simulink model "on_grid_new"  (R2015b)
settings: Solver=VariableStepAuto  StartTime=0.0  StopTime=5  RelTol=1e-3
undefined symbols (not defined in the file): Ts_Control, Ts_Power
libraries: powerlib x41, powerlib_meascontrol x16, simulink x3, powerlib_extras x1
settings Model: Creator=fujitsu  LastModifiedBy=fujitsu

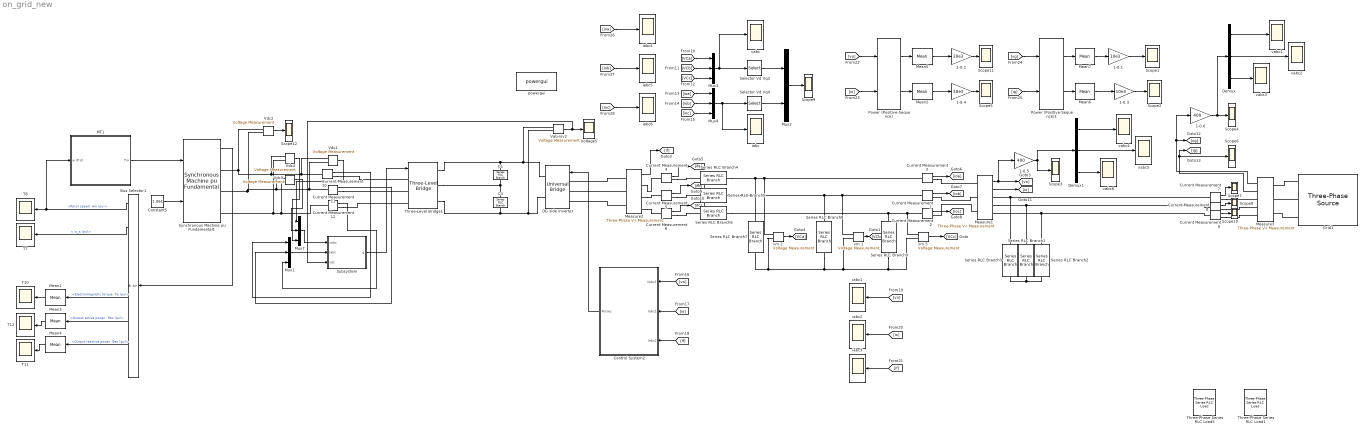
== system on_grid_new ==
  1-0.1 : Gain  Gain=10e3
  1-0.2 : Gain  Gain=30e3
  1-0.3 : Gain  Gain=10e3
  1-0.4 : Gain  Gain=30e3
  1-0.5 : Gain  Gain=400
  1-0.6 : Gain  Gain=400
  Bus Selector1 : BusSelector  OutputSignals="Mechanical.Rotor speed  wm (pu),Stator current. is_a (pu),Stator current. is_b (pu),Stator current. is_c (pu),Mechanical.Electromagnetic torque  Te (pu),Output active power   Peo (pu),Output reactive power  Qeo (pu),Mechanical.Rotor mechanical angle  theta (deg)"
  C1 : powerlib/Elements/Series RLC Branch  LConnTagsString=__new0  RConnTagsString=__new0  BranchType=C  Resistance=1.0  Inductance=1.0  SetiL0=off  InitialCurrent=0  Capacitance=5000e-06  Setx0=off  InitialVoltage=0  Measurements=None
  C3 : powerlib/Elements/Series RLC Branch  LConnTagsString=__new0  RConnTagsString=__new0  BranchType=C  Resistance=1.0  Inductance=1.0  SetiL0=off  InitialCurrent=0  Capacitance=5000e-06  Setx0=off  InitialVoltage=0  Measurements=None
  Constant5 : Constant  Value=1.061
  Control System2 : Subsystem
  Current Measurement{1..12} (12 alike) : powerlib/Measurements/Current Measurement  PhasorSimulation=off  OutputType=Complex  PSBequivalent=0
  DG side Inverter : powerlib/Power Electronics/Universal Bridge  Arms=3  SnubberResistance=10000  SnubberCapacitance=inf  Device=IGBT / Diodes  Ron=1e-4  Lon=0  ForwardVoltages="[  1  1  ]"  ForwardVoltage=.8  GTOparameters=[ 10e-6 , 20e-6 ]  IGBTparameters=[ 1e-6 , 2e-6 ]  Measurements=None  Measurements_2=None  converterType=Rectifier
  Demux : Demux  Outputs=3
  Demux1 : Demux  Outputs=3
  Grid1 : powerlib/Electrical Sources/Three-Phase Source  InternalConnection=Yg  VoltagePhases=off  Voltage=400  PhaseAngle=0  Voltage_phases=[25e3 25e3 25e3]/sqrt(3)  PhaseAngles_phases=[0 -120 +120]  Frequency=50  NonIdealSource=on  SpecifyImpedance=off  Resistance=0.02  Inductance=0.3e-3  ShortCircuitLevel=100e6  BaseVoltage=60e3  XRratio=1  BusType=swing  Pref=0  Qref=0  Prefabc=[10e3, 10e3, 10e3]  Qrefabc=[0, 0, 0]  Qmin=-inf  Qmax=inf
  MT1 : Subsystem
  Mean{1..7} (7 alike) : powerlib_meascontrol/Measurements/Mean  Freq=50  Vinit=0  Ts=5e-6
  Measure1 : powerlib/Measurements/Three-Phase V-I Measurement  VoltageMeasurement=phase-to-ground  SetLabelV=off  LabelV=V1  Vpu=on  VpuLL=off  CurrentMeasurement=yes  SetLabelI=off  LabelI=I1  Ipu=on  Pbase=30e3  Vbase=400  OutputType=Magnitude  PhasorSimulation=off  PSBequivalent=0
  Measure2 : powerlib/Measurements/Three-Phase V-I Measurement  VoltageMeasurement=no  SetLabelV=off  LabelV=V1  Vpu=off  VpuLL=off  CurrentMeasurement=yes  SetLabelI=off  LabelI=I1  Ipu=on  Pbase=30e3  Vbase=400  OutputType=Magnitude  PhasorSimulation=off  PSBequivalent=0
  Measure3 : powerlib/Measurements/Three-Phase V-I Measurement  VoltageMeasurement=phase-to-ground  SetLabelV=off  LabelV=V1  Vpu=on  VpuLL=off  CurrentMeasurement=yes  SetLabelI=off  LabelI=I1  Ipu=on  Pbase=10e3  Vbase=400  OutputType=Magnitude  PhasorSimulation=off  PSBequivalent=0
  Mux{1,3..4,7} (4 alike) : Mux  Inputs=3
  Mux2 : Mux  Inputs=2
  Power (Positive-Sequence) : powerlib_meascontrol/Measurements/Power (Positive-Sequence)  Freq=50  Vinit=[0, 0]  Iinit=[0, 0]  Ts=5e-6
  Power (Positive-Sequence)1 : powerlib_meascontrol/Measurements/Power (Positive-Sequence)  Freq=50  Vinit=[0, 0]  Iinit=[0, 0]  Ts=5e-6
  Scope{1..12} (12 alike) : Scope
  Selector Vd Vq3 : Selector  InputPortWidth=3  IndexOptions=Index vector (dialog)  Indices=[1]  OutputSizes=1
  Selector Vd Vq4 : Selector  InputPortWidth=3  IndexOptions=Index vector (dialog)  Indices=[1]  OutputSizes=1
  Series RLC Branch1 : powerlib/Elements/Series RLC Branch  LConnTagsString=__new0  RConnTagsString=__new0  BranchType=RL  Resistance=50*0.5  Inductance=100e-3*0.5  SetiL0=off  InitialCurrent=0  Capacitance=1e-6  Setx0=off  InitialVoltage=0  Measurements=None
  Series RLC Branch2 : powerlib/Elements/Series RLC Branch  LConnTagsString=__new0  RConnTagsString=__new0  BranchType=RL  Resistance=50*0.5  Inductance=100e-3*0.5  SetiL0=off  InitialCurrent=0  Capacitance=1e-6  Setx0=off  InitialVoltage=0  Measurements=None
  Series RLC Branch3 : powerlib/Elements/Series RLC Branch  LConnTagsString=__new0  RConnTagsString=__new0  BranchType=RL  Resistance=50*0.5  Inductance=100e-3*0.5  SetiL0=off  InitialCurrent=0  Capacitance=1e-6  Setx0=off  InitialVoltage=0  Measurements=None
  Series RLC Branch4 : powerlib/Elements/Series RLC Branch  LConnTagsString=__new0  RConnTagsString=__new0  BranchType=L  Resistance=5  Inductance=3e-3  SetiL0=off  InitialCurrent=0  Capacitance=1e-6  Setx0=off  InitialVoltage=0  Measurements=None
  Series RLC Branch5 : powerlib/Elements/Series RLC Branch  LConnTagsString=__new0  RConnTagsString=__new0  BranchType=L  Resistance=5  Inductance=3e-3  SetiL0=off  InitialCurrent=0  Capacitance=1e-6  Setx0=off  InitialVoltage=0  Measurements=None
  Series RLC Branch6 : powerlib/Elements/Series RLC Branch  LConnTagsString=__new0  RConnTagsString=__new0  BranchType=L  Resistance=5  Inductance=3e-3  SetiL0=off  InitialCurrent=0  Capacitance=1e-6  Setx0=off  InitialVoltage=0  Measurements=None
  Series RLC Branch7 : powerlib/Elements/Series RLC Branch  LConnTagsString=__new0  RConnTagsString=__new0  BranchType=C  Resistance=5  Inductance=10e-3  SetiL0=off  InitialCurrent=0  Capacitance=300e-6  Setx0=off  InitialVoltage=0  Measurements=None
  Series RLC Branch8 : powerlib/Elements/Series RLC Branch  LConnTagsString=__new0  RConnTagsString=__new0  BranchType=C  Resistance=5  Inductance=10e-3  SetiL0=off  InitialCurrent=0  Capacitance=300e-6  Setx0=off  InitialVoltage=0  Measurements=None
  Series RLC Branch9 : powerlib/Elements/Series RLC Branch  LConnTagsString=__new0  RConnTagsString=__new0  BranchType=C  Resistance=5  Inductance=10e-3  SetiL0=off  InitialCurrent=0  Capacitance=300e-6  Setx0=off  InitialVoltage=0  Measurements=None
  Subsystem : Subsystem  mask{kp=0.0001, ki=5, dcref=750}
      mask prompts: dcref "Vdc_ref"
  Synchronous Machine pu Fundamental1 : powerlib/Machines/Synchronous Machine pu Fundamental  PresetModel=No  MechanicalLoad=Mechanical power Pm  ShowDetailedParameters=on  RotorType=Salient-pole  Units=per unit fundamental parameters  MeasurementBus=off  NominalParameters="[ 30e3  550 1600]"  Stator="[ 0.2503  0.114  0.6875  0.6875 ]"  Field="[ 1  10e15/(100*pi)]"  Dampers2=[0.0652, 0.5134, 0.0287, 0.2553, 7.765e-3, 0.9167 ]  Dampers1="[ 1.17E-02  0.182  1.97E-02  0.384 ]"  Mechanical=[ 6 0 2]  PolePairs=20  InitialConditions="[ 0  0  0  0  0  0  0  0  1 ]"  SetSaturation=off  Saturation=[0.6404,0.7127,0.8441,0.9214,0.9956,1.082,1.19,1.316,1.457;0.7,0.7698,0.8872,0.9466,0.9969,1.046,1.1,1.151,1.201]  LoadFlowParameters=[1,0,0,0,0]  TsPowergui=0  TsBlock=-1  IterativeModel=Trapezoidal non iterative  BusType=swing  Pref=0  Qref=0  Qmin=-inf  Qmax=inf  PLF=0  QLF=0
  T{7..8,10..12} (5 alike) : Scope
  Three-Level Bridge1 : powerlib/Power Electronics/Three-Level Bridge  Arms=3  SnubberResistance=100  SbubberCapacitance=1e-6  Device=IGBT / Diodes  Ron=1e-3  ForwardVoltages=[350 1]  Measurements=All voltages and currents
  Three-Phase Series RLC Load1 : powerlib/Elements/Three-Phase Series RLC Load  LConnTagsString=A|B|C  Configuration=Y (grounded)  NominalVoltage=400  Vabc=[1e3 1e3 1e3]  Vabcp=[1e3 1e3 1e3]  NominalFrequency=50  UnbalancedPower=off  ActivePower=50e3  InductivePower=0  CapacitivePower=0  Pabc=[10e3 9e3 11e3]  QLabc=[100 90 110]  QCabc=[100 90 110]  Pabcp=[10e3 9e3 11e3]  QLabcp=[100 90 110]  QCabcp=[100 90 110]  Measurements=None  LoadType=constant Z
  Three-Phase Series RLC Load5 : powerlib/Elements/Three-Phase Series RLC Load  LConnTagsString=A|B|C  Configuration=Y (grounded)  NominalVoltage=400  Vabc=[1e3 1e3 1e3]  Vabcp=[1e3 1e3 1e3]  NominalFrequency=50  UnbalancedPower=off  ActivePower=50e3  InductivePower=0  CapacitivePower=0  Pabc=[10e3 9e3 11e3]  QLabc=[100 90 110]  QCabc=[100 90 110]  Pabcp=[10e3 9e3 11e3]  QLabcp=[100 90 110]  QCabcp=[100 90 110]  Measurements=None  LoadType=constant Z
  Vab-inv2 : powerlib/Measurements/Voltage Measurement  Tag=PoWeRsYsTeMmEaSuReMeNt  PhasorSimulation=off  OutputType=Magnitude  PSBequivalent=0
  Vdc{1..4} (4 alike) : powerlib/Measurements/Voltage Measurement  Tag=PoWeRsYsTeMmEaSuReMeNt  PhasorSimulation=off  OutputType=Magnitude  PSBequivalent=0
  Voltage5 : Scope
  iabc{,1..6} (7 alike) : Scope
  powergui : powerlib/powergui  SimulationMode=Discrete  SolverType=Tustin  SampleTime=5e-6  frequency=60  SPID=off  DisableSnubberDevices=off  DisableRonSwitches=off  DisableVfSwitches=off  SwTol=0  DisplayEquations=off  Interpol=off  ExternalGateDelay=off  methode=off  Ts=0  FunctionMessages=off  echomessages=off  HookPort=off  EnableUseOfTLC=off  x0status=blocks  frequencyindice=0  Pbase=100e6  ErrMax=0.0001  Iterations=50  UnitsV=kV  UnitsW=MW  buscounter=0  RestoreLinks=warning  ResistiveCurrentMeasurement=off  Frange=[0:2:500]  Ylog=off  Xlog=on  ShowGrid=off  save=off  variable=ZData  structure=Vs  ZoomFFT=on  StartTime=1/60  cycles=1  DisplayStyle=1  fundamental=60  FreqAxis=on  MaxFrequency=10000  frequencyindicesteady=1  RmsSteady=1  display=off
  vabc{,1..6} (7 alike) : Scope
  vm 1 : powerlib/Measurements/Voltage Measurement  PhasorSimulation=off  OutputType=Complex  PSBequivalent=0
  vm 2 : powerlib/Measurements/Voltage Measurement  PhasorSimulation=off  OutputType=Complex  PSBequivalent=0
  vm 5 : powerlib/Measurements/Voltage Measurement  PhasorSimulation=off  OutputType=Complex  PSBequivalent=0
  wires:
  Control System2/1(Pulses) -> DG side Inverter/1
  vm 5/1 -> [VCc]
  vm 1/1 -> [VCb]
  vm 2/1 -> [VCa]
  Current Measurement2/1 -> [ioc]
  Current Measurement1/1 -> [iob]
  Current Measurement3/1 -> [ioa]
  Current Measurement4/1 -> [ifa]
  Current Measurement5/1 -> [ifb]
  Current Measurement6/1 -> [ifc]
  Power (Positive-Sequence)/1 -> Mean5/1
  Mux2/1 -> Scope9/1
  Selector Vd Vq3/1 -> Mux2/1
  Selector Vd Vq4/1 -> Mux2/2
  Power (Positive-Sequence)/2 -> Mean2/1
  [VCc] -> Mux3/3
  [VCa] -> Mux3/1
  [VCb] -> Mux3/2
  Mux3/1 -> Selector Vd Vq3/1, vabc/1
  [ioa] -> Mux4/1
  [iob] -> Mux4/2
  [ioc] -> Mux4/3
  Mux4/1 -> Selector Vd Vq4/1, iabc/1
  Measure2/1 -> [if]
  Measure1/1 -> 1-0.5/1, [vo]
  Measure1/2 -> [io]
  [vo] -> Control System2/1(Vabc1)
  [vo] -> iabc1/1
  [io] -> iabc2/1
  [if] -> iabc3/1
  Measure3/1 -> 1-0.6/1, [vg]
  Measure3/2 -> [ig], Scope6/1
  Power (Positive-Sequence)1/1 -> Mean7/1
  Power (Positive-Sequence)1/2 -> Mean6/1
  [vg] -> Power (Positive-Sequence)1/1
  [ig] -> Power (Positive-Sequence)1/2
  Mean7/1 -> 1-0.1/1
  Mean6/1 -> 1-0.3/1
  1-0.3/1 -> Scope2/1
  1-0.1/1 -> Scope1/1
  1-0.2/1 -> Scope11/1
  Mean5/1 -> 1-0.2/1
  1-0.4/1 -> Scope5/1
  Mean2/1 -> 1-0.4/1
  [io] -> Control System2/2(Iabc1)
  [if] -> Control System2/3(Iabc2)
  1-0.5/1 -> Demux1/1, Scope3/1
  1-0.6/1 -> Demux/1, Scope4/1
  [ioa] -> iabc4/1
  [iob] -> iabc5/1
  [ioc] -> iabc6/1
  Demux/3 -> vabc3/1
  Demux/2 -> vabc2/1
  Demux/1 -> vabc1/1
  [vo] -> Power (Positive-Sequence)/1
  [io] -> Power (Positive-Sequence)/2
  Demux1/3 -> vabc6/1
  Demux1/2 -> vabc5/1
  Demux1/1 -> vabc4/1
  Current Measurement7/1 -> Scope7/1
  Current Measurement8/1 -> Scope8/1
  Current Measurement9/1 -> Scope10/1
  MT1/1(Tm) -> Synchronous Machine pu Fundamental1/1
  Synchronous Machine pu Fundamental1/1 -> Bus Selector1/1
  Constant5/1 -> Synchronous Machine pu Fundamental1/2
  Vdc2/1 -> Scope12/1
  Vab-inv2/1 -> Subsystem/3(vdc), Voltage5/1
  Mean4/1 -> T11/1
  Bus Selector1/1 -> MT1/1(w (P.U)), T8/1  "<Rotor speed  wm (pu)>"
  Bus Selector1/5 -> Mean1/1  "<Electromagnetic torque  Te (pu)>"
  Mean1/1 -> T10/1
  Bus Selector1/7 -> Mean4/1  "<Output reactive power  Qeo (pu)>"
  Bus Selector1/6 -> Mean3/1  "<Output active power   Peo (pu)>"
  Mean3/1 -> T12/1
  Bus Selector1/2 -> T7/1  "< is_a (pu)>"
  Subsystem/1(g) -> Three-Level Bridge1/1
  Current Measurement10/1 -> Mux1/1
  Current Measurement11/1 -> Mux1/2
  Current Measurement12/1 -> Mux1/3
  Mux1/1 -> Subsystem/2(Iabc)
  Vdc1/1 -> Mux7/1
  Vdc3/1 -> Mux7/2
  Vdc4/1 -> Mux7/3
  Mux7/1 -> Subsystem/1(vabc)
  connections:
  C3/RConn1 -- Three-Level Bridge1/RConn3 -- DG side Inverter/RConn2 -- Vab-inv2/LConn2
  Three-Level Bridge1/RConn1 -- C1/LConn1 -- DG side Inverter/RConn1 -- Vab-inv2/LConn1
  Series RLC Branch7/LConn1 -- Series RLC Branch4/RConn1 -- Current Measurement3/LConn1 -- vm 2/LConn1
  Current Measurement1/LConn1 -- vm 1/LConn1 -- Series RLC Branch5/RConn1 -- Series RLC Branch8/LConn1
  Series RLC Branch9/LConn1 -- Series RLC Branch6/RConn1 -- Current Measurement2/LConn1 -- vm 5/LConn1
  vm 2/LConn2 -- Series RLC Branch7/RConn1 -- Series RLC Branch8/RConn1 -- vm 1/LConn2 -- Series RLC Branch9/RConn1 -- vm 5/LConn2
  Measure1/RConn1 -- Current Measurement7/LConn1 -- Series RLC Branch3/LConn1
  Measure1/RConn3 -- Current Measurement9/LConn1 -- Series RLC Branch2/LConn1
  Series RLC Branch1/LConn1 -- Current Measurement8/LConn1 -- Measure1/RConn2
  Series RLC Branch2/RConn1 -- Series RLC Branch3/RConn1 -- Series RLC Branch1/RConn1
  Current Measurement8/RConn1 -- Measure3/RConn2
  Measure2/RConn3 -- Current Measurement6/LConn1
  Current Measurement9/RConn1 -- Measure3/RConn3
  Grid1/RConn1 -- Measure3/LConn1
  Measure2/LConn3 -- DG side Inverter/LConn3
  Measure2/RConn2 -- Current Measurement5/LConn1
  Grid1/RConn2 -- Measure3/LConn2
  Current Measurement6/RConn1 -- Series RLC Branch6/LConn1
  Measure2/RConn1 -- Current Measurement4/LConn1
  Current Measurement4/RConn1 -- Series RLC Branch4/LConn1
  Current Measurement5/RConn1 -- Series RLC Branch5/LConn1
  Measure1/LConn3 -- Current Measurement2/RConn1
  Current Measurement7/RConn1 -- Measure3/RConn1
  Grid1/RConn3 -- Measure3/LConn3
  Current Measurement3/RConn1 -- Measure1/LConn1
  Measure2/LConn2 -- DG side Inverter/LConn2
  Measure1/LConn2 -- Current Measurement1/RConn1
  Measure2/LConn1 -- DG side Inverter/LConn1
  Synchronous Machine pu Fundamental1/RConn2 -- Vdc2/LConn2 -- Vdc3/LConn1 -- Vdc1/LConn2 -- Current Measurement11/LConn1
  C1/RConn1 -- Three-Level Bridge1/RConn2 -- C3/LConn1
  Synchronous Machine pu Fundamental1/RConn1 -- Vdc2/LConn1 -- Vdc4/LConn1 -- Vdc1/LConn1 -- Current Measurement10/LConn1
  Synchronous Machine pu Fundamental1/RConn3 -- Vdc4/LConn2 -- Current Measurement12/LConn1 -- Vdc3/LConn2
  Current Measurement11/RConn1 -- Three-Level Bridge1/LConn2
  Current Measurement12/RConn1 -- Three-Level Bridge1/LConn3
  Current Measurement10/RConn1 -- Three-Level Bridge1/LConn1

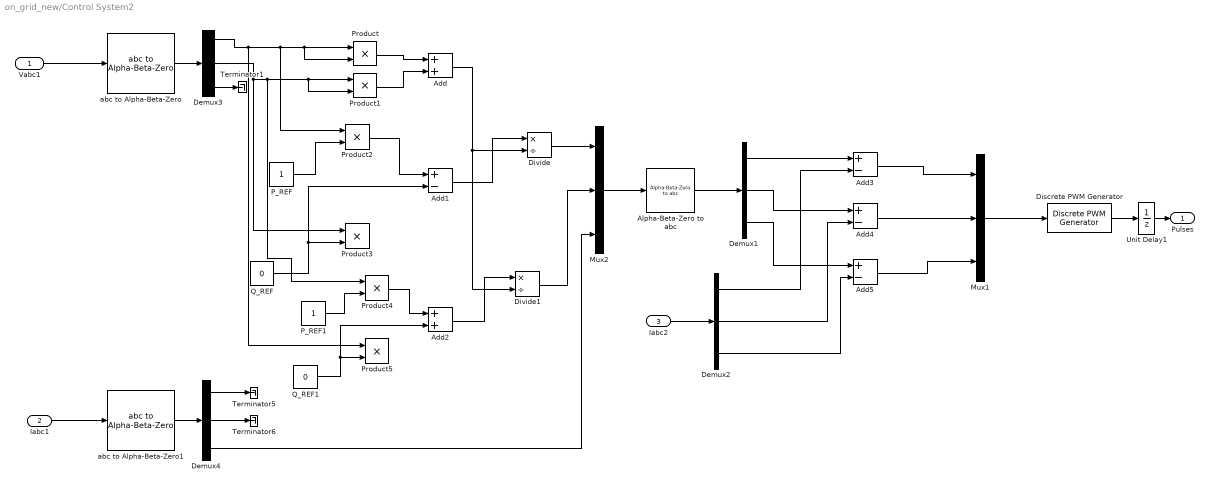
== system on_grid_new/Control System2 ==
  Vabc1 : Inport  PortDimensions=3
  Iabc1 : Inport  Port=2  PortDimensions=3
  Iabc2 : Inport  Port=3  PortDimensions=3
  Add : Sum
  Add{1,3..5} (4 alike) : Sum  Inputs=+-
  Add2 : Sum
  Alpha-Beta-Zero to abc : powerlib_meascontrol/Transformations/Alpha-Beta-Zero to abc
  Demux{1..4} (4 alike) : Demux  Outputs=3
  Discrete PWM Generator : powerlib_extras/Discrete  Control Blocks/Discrete PWM Generator  GeneratorMode="3-arm  bridge (6 pulses)"  Fc=8000  Ts=5e-6  Internal=off  mIndex=0.4  Freq=60  Phase=0
  Divide : Product  Inputs=*/
  Divide1 : Product  Inputs=*/
  Mux1 : Mux  Inputs=3
  Mux2 : Mux  Inputs=3
  P_REF : Constant
  P_REF1 : Constant
  Product{,1..5} (6 alike) : Product
  Q_REF : Constant  Value=0
  Q_REF1 : Constant  Value=0
  Terminator1 : Terminator
  Terminator5 : Terminator
  Terminator6 : Terminator
  Unit Delay1 : UnitDelay  SampleTime=5e-6
  abc to Alpha-Beta-Zero : powerlib_meascontrol/Transformations/abc to Alpha-Beta-Zero
  abc to Alpha-Beta-Zero1 : powerlib_meascontrol/Transformations/abc to Alpha-Beta-Zero
  Pulses : Outport
  wires:
  Unit Delay1/1 -> Pulses/1
  Discrete PWM Generator/1 -> Unit Delay1/1
  Vabc1/1 -> abc to Alpha-Beta-Zero/1
  abc to Alpha-Beta-Zero/1 -> Demux3/1
  Demux3/1 -> Product/1, Product/2, Product2/1, Product5/1
  Demux3/2 -> Product4/1, Product1/2, Product1/1, Product3/1
  Product/1 -> Add/1
  Product1/1 -> Add/2
  P_REF/1 -> Product2/2
  Q_REF/1 -> Add1/2, Product3/2
  Product2/1 -> Add1/1
  Add1/1 -> Divide/1
  Add/1 -> Divide1/2, Divide/2
  Divide/1 -> Mux2/1
  P_REF1/1 -> Product4/2
  Q_REF1/1 -> Add2/2, Product5/2
  Product4/1 -> Add2/1
  Add2/1 -> Divide1/1
  Divide1/1 -> Mux2/2
  Iabc1/1 -> abc to Alpha-Beta-Zero1/1
  abc to Alpha-Beta-Zero1/1 -> Demux4/1
  Demux4/3 -> Mux2/3
  Demux4/1 -> Terminator5/1
  Demux4/2 -> Terminator6/1
  Mux2/1 -> Alpha-Beta-Zero to abc/1
  Alpha-Beta-Zero to abc/1 -> Demux1/1
  Demux1/1 -> Add3/1
  Iabc2/1 -> Demux2/1
  Demux2/1 -> Add3/2
  Demux1/2 -> Add4/1
  Demux2/2 -> Add4/2
  Demux1/3 -> Add5/1
  Demux2/3 -> Add5/2
  Add3/1 -> Mux1/1
  Add4/1 -> Mux1/2
  Add5/1 -> Mux1/3
  Mux1/1 -> Discrete PWM Generator/1
  Demux3/3 -> Terminator1/1

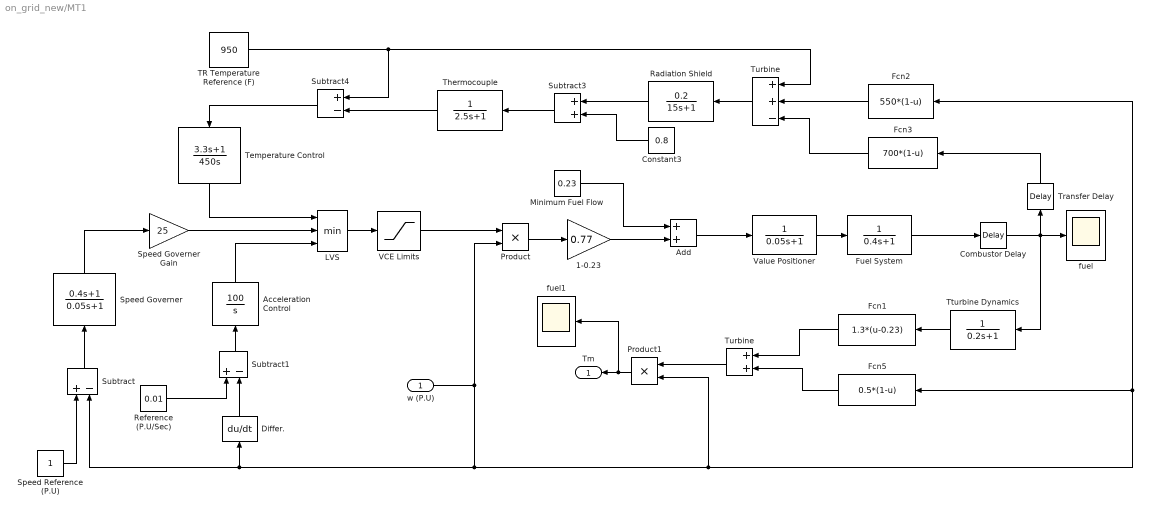
== system on_grid_new/MT1 ==
  w (P.U) : Inport
  1-0.23 : Gain  Gain=0.77
  Acceleration Control : TransferFcn  Numerator=[0 100]  Denominator=[1 0]
  Add : Sum
  Combustor Delay : TransportDelay  DelayTime=0.01
  Constant3 : Constant  Value=0.8
  Differ. : Derivative
  Fcn1 : Fcn  Expr=1.3*(u-0.23)
  Fcn2 : Fcn  Expr=550*(1-u)
  Fcn3 : Fcn  Expr=700*(1-u)
  Fcn5 : Fcn  Expr=0.5*(1-u)
  Fuel System : TransferFcn  Denominator=[0.4 1]
  LVS : MinMax  Inputs=3
  Minimum Fuel Flow : Constant  Value=0.23
  Product : Product  RndMeth=Zero
  Product1 : Product  RndMeth=Zero
  Radiation Shield : TransferFcn  Numerator=[0.2]  Denominator=[15 1]
  Reference (P.U/Sec) : Constant  Value=0.01
  Speed Governer : TransferFcn  Numerator=[0.4 1]  Denominator=[0.05 1]
  Speed Governer Gain : Gain  Gain=25
  Speed Reference (P.U) : Constant
  Subtract : Sum  Inputs=+-
  Subtract1 : Sum  Inputs=+-
  Subtract3 : Sum
  Subtract4 : Sum  Inputs=+-
  TR Temperature Reference (F) : Constant  Value=950
  Temperature Control : TransferFcn  Numerator=[3.3 1]  Denominator=[450 0]
  Thermocouple : TransferFcn  Denominator=[2.5 1]
  Transfer Delay : TransportDelay  DelayTime=0.04
  Tturbine Dynamics : TransferFcn  Denominator=[0.2 1]
  Turbine : Sum  Inputs=++-
  "Turbine " : Sum
  VCE Limits : Saturate  UpperLimit=1.5  LowerLimit=-0.1
  Value Positioner : TransferFcn  Denominator=[0.05 1]
  fuel : Scope
  fuel1 : Scope
  Tm : Outport
  wires:
  "Turbine "/1 -> Product1/1
  Product1/1 -> fuel1/1, Tm/1
  Fcn5/1 -> "Turbine "/2
  Fcn1/1 -> "Turbine "/1
  Tturbine Dynamics/1 -> Fcn1/1
  w (P.U)/1 -> Fcn2/1, Fcn5/1, Product1/2, Differ./1, Subtract/2, Product/2
  Speed Governer/1 -> Speed Governer Gain/1
  Temperature Control/1 -> LVS/1
  Subtract4/1 -> Temperature Control/1
  TR Temperature Reference (F)/1 -> Subtract4/1, Turbine/1
  Thermocouple/1 -> Subtract4/2
  Subtract3/1 -> Thermocouple/1
  Turbine/1 -> Radiation Shield/1
  Constant3/1 -> Subtract3/2
  Radiation Shield/1 -> Subtract3/1
  Fcn2/1 -> Turbine/2
  Fcn3/1 -> Turbine/3
  Transfer Delay/1 -> Fcn3/1
  LVS/1 -> VCE Limits/1
  Acceleration Control/1 -> LVS/3
  Subtract1/1 -> Acceleration Control/1
  Reference (P.U/Sec)/1 -> Subtract1/1
  Differ./1 -> Subtract1/2
  Speed Governer Gain/1 -> LVS/2
  Combustor Delay/1 -> Tturbine Dynamics/1, fuel/1, Transfer Delay/1
  Fuel System/1 -> Combustor Delay/1
  Value Positioner/1 -> Fuel System/1
  Add/1 -> Value Positioner/1
  Minimum Fuel Flow/1 -> Add/1
  1-0.23/1 -> Add/2
  Product/1 -> 1-0.23/1
  VCE Limits/1 -> Product/1
  Subtract/1 -> Speed Governer/1
  Speed Reference (P.U)/1 -> Subtract/1

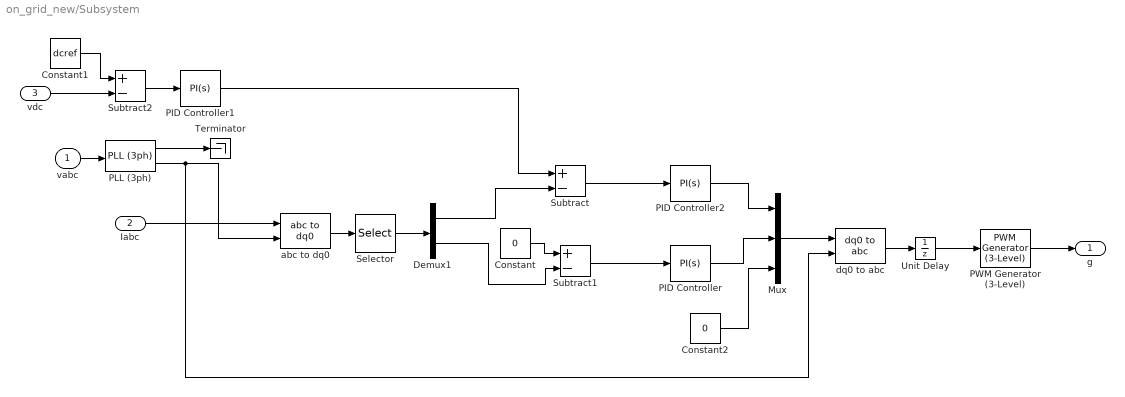
== system on_grid_new/Subsystem ==
  vabc : Inport
  Iabc : Inport  Port=2
  vdc : Inport  Port=3
  Constant : Constant  Value=0
  Constant1 : Constant  Value=dcref
  Constant2 : Constant  Value=0
  Demux1 : Demux  Outputs=2
  Mux : Mux  Inputs=3
  PID Controller : simulink/Continuous/PID Controller  Controller=PI  TimeDomain=Continuous-time  SampleTime=-1  IntegratorMethod=Forward Euler  FilterMethod=Forward Euler  Form=Parallel  UseFilter=on  ControllerParametersSource=internal  P=kp  I=ki  D=0  N=100  InitialConditionSource=internal  InitialConditionForIntegrator=0  InitialConditionForFilter=0  ExternalReset=none  LimitOutput=off  UpperSaturationLimit=inf  LowerSaturationLimit=-inf  LinearizeAsGain=on  AntiWindupMode=none  Kb=1  TrackingMode=off  Kt=1  PParamMin=[]  PParamMax=[]  IParamMin=[]  IParamMax=[]  DParamMin=[]  DParamMax=[]  NParamMin=[]  NParamMax=[]  KbParamMin=[]  KbParamMax=[]  KtParamMin=[]  KtParamMax=[]  POutMin=[]  POutMax=[]  IOutMin=[]  IOutMax=[]  DOutMin=[]  DOutMax=[]  NOutMin=[]  NOutMax=[]  KbOutMin=[]  KbOutMax=[]  KtOutMin=[]  KtOutMax=[]  IntegratorOutMin=[]  IntegratorOutMax=[]  FilterOutMin=[]  FilterOutMax=[]  SumOutMin=[]  SumOutMax=[]  SumI1OutMin=[]  SumI1OutMax=[]  SumI2OutMin=[]  SumI2OutMax=[]  SumI3OutMin=[]  SumI3OutMax=[]  SumDOutMin=[]  SumDOutMax=[]  SaturationOutMin=[]  SaturationOutMax=[]  IntegratorContinuousStateAttributes=''  IntegratorStateMustResolveToSignalObject=off  IntegratorRTWStateStorageClass=Auto  FilterContinuousStateAttributes=''  FilterStateMustResolveToSignalObject=off  FilterRTWStateStorageClass=Auto  DifferentiatorICPrevScaledInput=0  DifferentiatorOutMin=[]  DifferentiatorOutMax=[]
  PID Controller1 : simulink/Continuous/PID Controller  Controller=PI  TimeDomain=Continuous-time  SampleTime=-1  IntegratorMethod=Forward Euler  FilterMethod=Forward Euler  Form=Parallel  UseFilter=on  ControllerParametersSource=internal  P=kp  I=ki  D=0  N=100  InitialConditionSource=internal  InitialConditionForIntegrator=0  InitialConditionForFilter=0  ExternalReset=none  LimitOutput=off  UpperSaturationLimit=inf  LowerSaturationLimit=-inf  LinearizeAsGain=on  AntiWindupMode=none  Kb=1  TrackingMode=off  Kt=1  PParamMin=[]  PParamMax=[]  IParamMin=[]  IParamMax=[]  DParamMin=[]  DParamMax=[]  NParamMin=[]  NParamMax=[]  KbParamMin=[]  KbParamMax=[]  KtParamMin=[]  KtParamMax=[]  POutMin=[]  POutMax=[]  IOutMin=[]  IOutMax=[]  DOutMin=[]  DOutMax=[]  NOutMin=[]  NOutMax=[]  KbOutMin=[]  KbOutMax=[]  KtOutMin=[]  KtOutMax=[]  IntegratorOutMin=[]  IntegratorOutMax=[]  FilterOutMin=[]  FilterOutMax=[]  SumOutMin=[]  SumOutMax=[]  SumI1OutMin=[]  SumI1OutMax=[]  SumI2OutMin=[]  SumI2OutMax=[]  SumI3OutMin=[]  SumI3OutMax=[]  SumDOutMin=[]  SumDOutMax=[]  SaturationOutMin=[]  SaturationOutMax=[]  IntegratorContinuousStateAttributes=''  IntegratorStateMustResolveToSignalObject=off  IntegratorRTWStateStorageClass=Auto  FilterContinuousStateAttributes=''  FilterStateMustResolveToSignalObject=off  FilterRTWStateStorageClass=Auto  DifferentiatorICPrevScaledInput=0  DifferentiatorOutMin=[]  DifferentiatorOutMax=[]
  PID Controller2 : simulink/Continuous/PID Controller  Controller=PI  TimeDomain=Continuous-time  SampleTime=-1  IntegratorMethod=Forward Euler  FilterMethod=Forward Euler  Form=Parallel  UseFilter=on  ControllerParametersSource=internal  P=kp  I=ki  D=0  N=100  InitialConditionSource=internal  InitialConditionForIntegrator=0  InitialConditionForFilter=0  ExternalReset=none  LimitOutput=off  UpperSaturationLimit=inf  LowerSaturationLimit=-inf  LinearizeAsGain=on  AntiWindupMode=none  Kb=1  TrackingMode=off  Kt=1  PParamMin=[]  PParamMax=[]  IParamMin=[]  IParamMax=[]  DParamMin=[]  DParamMax=[]  NParamMin=[]  NParamMax=[]  KbParamMin=[]  KbParamMax=[]  KtParamMin=[]  KtParamMax=[]  POutMin=[]  POutMax=[]  IOutMin=[]  IOutMax=[]  DOutMin=[]  DOutMax=[]  NOutMin=[]  NOutMax=[]  KbOutMin=[]  KbOutMax=[]  KtOutMin=[]  KtOutMax=[]  IntegratorOutMin=[]  IntegratorOutMax=[]  FilterOutMin=[]  FilterOutMax=[]  SumOutMin=[]  SumOutMax=[]  SumI1OutMin=[]  SumI1OutMax=[]  SumI2OutMin=[]  SumI2OutMax=[]  SumI3OutMin=[]  SumI3OutMax=[]  SumDOutMin=[]  SumDOutMax=[]  SaturationOutMin=[]  SaturationOutMax=[]  IntegratorContinuousStateAttributes=''  IntegratorStateMustResolveToSignalObject=off  IntegratorRTWStateStorageClass=Auto  FilterContinuousStateAttributes=''  FilterStateMustResolveToSignalObject=off  FilterRTWStateStorageClass=Auto  DifferentiatorICPrevScaledInput=0  DifferentiatorOutMin=[]  DifferentiatorOutMax=[]
  PLL (3ph) : powerlib_meascontrol/PLL/PLL (3ph)  Fmin=45  Par_Init=[0, 50]  ParK=[180, 3200, 1]  TcD=1e-4  MaxRateChangeFreq=12  FilterCutOffFreq=25  Ts=0  AGC=on
  PWM Generator (3-Level) : powerlib_meascontrol/Pulse & Signal Generators/PWM Generator (3-Level)  ModulatorType=Three-phase bridge (12 pulses)  ModulatorMode=Unsynchronized  nF=27  Fc=1e3  ModulatingSignals=off  m=0.8  Freq=60  Phase=0  Ts=Ts_Power
  Selector : Selector  InputPortWidth=3  IndexOptions=Index vector (dialog)  Indices=[1 2]  OutputSizes=1
  Subtract : Sum  Inputs=+-
  Subtract1 : Sum  Inputs=+-
  Subtract2 : Sum  Inputs=+-
  Terminator : Terminator
  Unit Delay : UnitDelay  SampleTime=Ts_Control
  abc to dq0 : powerlib_meascontrol/Transformations/abc to dq0  Alignment=90 degrees behind phase A axis
  dq0 to abc : powerlib_meascontrol/Transformations/dq0 to abc  Alignment=90 degrees behind phase A axis
  g : Outport
  wires:
  vabc/1 -> PLL (3ph)/1
  PLL (3ph)/2 -> dq0 to abc/2, abc to dq0/2
  Iabc/1 -> abc to dq0/1
  PLL (3ph)/1 -> Terminator/1
  abc to dq0/1 -> Selector/1
  Selector/1 -> Demux1/1
  Demux1/1 -> Subtract/2
  Demux1/2 -> Subtract1/2
  Constant/1 -> Subtract1/1
  Subtract1/1 -> PID Controller/1
  vdc/1 -> Subtract2/2
  Constant1/1 -> Subtract2/1
  Subtract2/1 -> PID Controller1/1
  PID Controller1/1 -> Subtract/1
  Subtract/1 -> PID Controller2/1
  PID Controller2/1 -> Mux/1
  PID Controller/1 -> Mux/2
  Constant2/1 -> Mux/3
  Mux/1 -> dq0 to abc/1
  dq0 to abc/1 -> Unit Delay/1
  PWM Generator (3-Level)/1 -> g/1
  Unit Delay/1 -> PWM Generator (3-Level)/1
